simulink model "Subsystem1"  (R2023b)
settings: Solver=FixedStepAuto  StartTime=0.0  StopTime=10.0  FixedStep=5e-7  RelTol=1e-3
libraries: spsMosfetLib x6, spsDCVoltageSourceLib x1, spsPermanentMagnetSynchronousMachineLib x1, sps_lib x1
settings Model: Creator=LZQ  LastModifiedBy=LZQ
settings SolverCC: AllowMultiTaskInputOutput=on  ConcurrentTasks=on
settings DataIOCC: SaveOutput=off  SaveTime=off

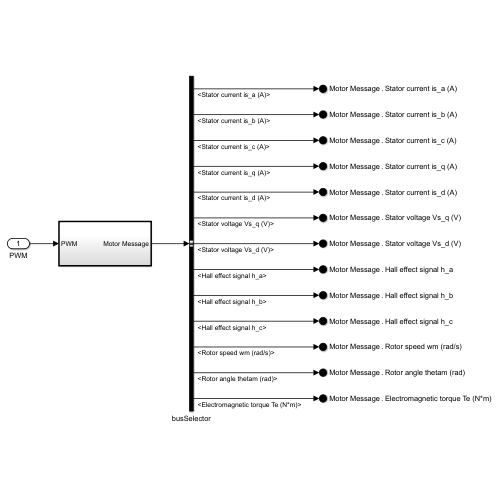
[thumbnail: Simulink's stored preview of the top-level diagram]
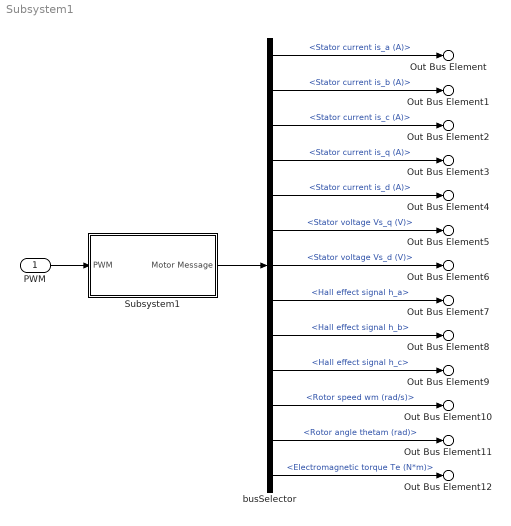
== system Subsystem1 ==
  PWM : Inport  OutDataTypeStr=double  PortDimensions=6  SampleTime=0
  Subsystem1 : Subsystem  TreatAsAtomicUnit=on
  busSelector : BusSelector  OutputSignals=Stator current is_a (A),Stator current is_b (A),Stator current is_c (A),Stator current is_q (A),Stator current is_d (A),Stator voltage Vs_q (V),Stator voltage Vs_d (V),Hall effect signal h_a,Hall effect signal h_b,Hall effect signal h_c,Rotor speed wm (rad/s),Rotor angle thetam (rad),Electromagnetic torque Te (N*m)
  Out Bus Element : Outport  PortName=Motor Message  Element=Stator current is_a (A)
  Out Bus Element1 : Outport  PortName=Motor Message  Element=Stator current is_b (A)
  Out Bus Element2 : Outport  PortName=Motor Message  Element=Stator current is_c (A)
  Out Bus Element3 : Outport  PortName=Motor Message  Element=Stator current is_q (A)
  Out Bus Element4 : Outport  PortName=Motor Message  Element=Stator current is_d (A)
  Out Bus Element5 : Outport  PortName=Motor Message  Element=Stator voltage Vs_q (V)
  Out Bus Element6 : Outport  PortName=Motor Message  Element=Stator voltage Vs_d (V)
  Out Bus Element7 : Outport  PortName=Motor Message  Element=Hall effect signal h_a
  Out Bus Element8 : Outport  PortName=Motor Message  Element=Hall effect signal h_b
  Out Bus Element9 : Outport  PortName=Motor Message  Element=Hall effect signal h_c
  Out Bus Element10 : Outport  PortName=Motor Message  Element=Rotor speed wm (rad/s)
  Out Bus Element11 : Outport  PortName=Motor Message  Element=Rotor angle thetam (rad)
  Out Bus Element12 : Outport  PortName=Motor Message  Element=Electromagnetic torque Te (N*m)
  wires:
  busSelector/4 -> Out Bus Element3/1  "<Stator current is_q (A)>"
  PWM/1 -> Subsystem1/1(PWM)
  busSelector/2 -> Out Bus Element1/1  "<Stator current is_b (A)>"
  Subsystem1/1(Motor Message) -> busSelector/1
  busSelector/1 -> Out Bus Element/1  "<Stator current is_a (A)>"
  busSelector/3 -> Out Bus Element2/1  "<Stator current is_c (A)>"
  busSelector/5 -> Out Bus Element4/1  "<Stator current is_d (A)>"
  busSelector/6 -> Out Bus Element5/1  "<Stator voltage Vs_q (V)>"
  busSelector/7 -> Out Bus Element6/1  "<Stator voltage Vs_d (V)>"
  busSelector/8 -> Out Bus Element7/1  "<Hall effect signal h_a>"
  busSelector/9 -> Out Bus Element8/1  "<Hall effect signal h_b>"
  busSelector/10 -> Out Bus Element9/1  "<Hall effect signal h_c>"
  busSelector/11 -> Out Bus Element10/1  "<Rotor speed wm (rad/s)>"
  busSelector/12 -> Out Bus Element11/1  "<Rotor angle thetam (rad)>"
  busSelector/13 -> Out Bus Element12/1  "<Electromagnetic torque Te (N*m)>"

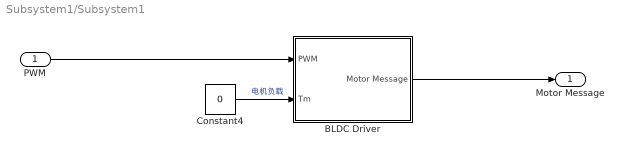
== system Subsystem1/Subsystem1 ==
  PWM : Inport
  BLDC Driver : Subsystem
  Constant4 : Constant  Value=0
  Motor Message : Outport
  wires:
  BLDC Driver/1(Motor Message) -> Motor Message/1
  PWM/1 -> BLDC Driver/1(PWM)
  Constant4/1 -> BLDC Driver/2(Tm)  "电机负载"

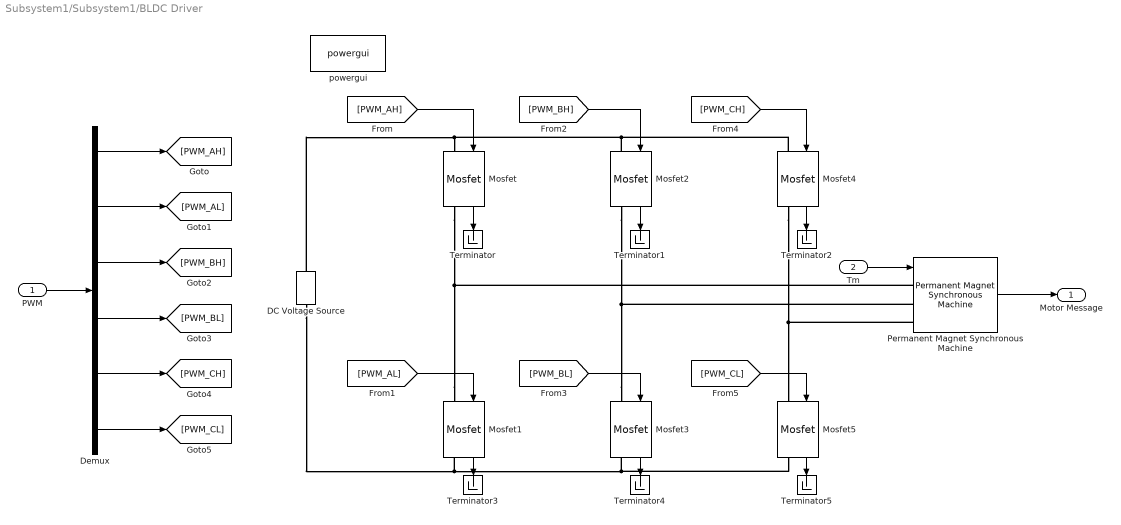
== system Subsystem1/Subsystem1/BLDC Driver ==
  PWM : Inport
  Tm : Inport  Port=2
  DC Voltage Source : spsDCVoltageSourceLib/DC Voltage Source  Amplitude=100  Measurements=Voltage
  Demux : Demux  Outputs=6
  Mosfet{,1..5} (6 alike) : spsMosfetLib/Mosfet  Ron=0.1  Lon=0  Rd=0.01  Vfd=0  IC=0  Rs=1e5  Cs=inf  Measurements=on
  Permanent Magnet Synchronous Machine : spsPermanentMagnetSynchronousMachineLib/Permanent Magnet Synchronous Machine  NbPhases=3  FluxDistribution=Sinusoidal  RotorType=Round  MechanicalLoad=Torque Tm  PresetModel=No  ShowDetailedParameters=on  MeasurementBus=off  Resistance=0.0485  Inductance=8.5e-3  dqInductances=[8.5e-3,8.5e-3]  La=0.000395  MachineConstant=Flux linkage established by magnets (V.s)  Flux=0.1194  VoltageCst=86.6271  TorqueCst=0.7164  Flat=120  Mechanical=[0.0027 0.0004924 4 0]  PolePairs=4  InitialConditions=[0,0, 0,0]  InitialConditions5ph=[0 0 0 0 0 0]  RefAngle=90 degrees behind phase A axis (modified Park)  IterativeDiscreteModel=Trapezoidal non iterative  TsBlock=-1  TsPowergui=0
  Terminator{,1..5} (6 alike) : Terminator
  powergui : sps_lib/powergui  Priority=1  SimulationMode=Discrete  SampleTime=5e-7  frequency=60  Iterations=50  frequencyindice=0  Pbase=100e6  ErrMax=1e-4  UnitsV=kV  UnitsW=MW  buscounter=0  FunctionMessages=off  echomessages=off  EnableUseOfTLC=off  CurrentSourceSwitches=off  DisableSnubberDevices=off  DisableRonSwitches=off  DisableVfSwitches=off  DisplayEquations=off  AutomaticDiscreteSolvers=off  SolverType=Tustin/Backward Euler (TBE)  Interpol=off  ExternalGateDelay=off  methode=off  Ts=100  x0status=blocks  SPID=on  SwTol=0  HookPort=off  NonlinearTolerance=1e-4  nMaxIteration=100  ContinueOnMaxIteration=off  RestoreLinks=warning  ResistiveCurrentMeasurement=off  Frange=[0:2:500]  Ylog=off  Xlog=on  ShowGrid=off  save=off  variable=ZData  structure=0  ZoomFFT=off  StartTime=0.0  cycles=1  DisplayStyle=1  fundamental=60  FreqAxis=off  MaxFrequency=1000  frequencyindicesteady=1  RmsSteady=1  display=off
  Motor Message : Outport
  wires:
  Tm/1 -> Permanent Magnet Synchronous Machine/1
  Permanent Magnet Synchronous Machine/1 -> Motor Message/1
  Demux/6 -> [PWM_CL]
  Demux/5 -> [PWM_CH]
  Demux/4 -> [PWM_BL]
  Demux/3 -> [PWM_BH]
  Demux/2 -> [PWM_AL]
  Demux/1 -> [PWM_AH]
  PWM/1 -> Demux/1
  [PWM_CL] -> Mosfet5/1
  [PWM_CH] -> Mosfet4/1
  [PWM_AL] -> Mosfet1/1
  [PWM_BL] -> Mosfet3/1
  [PWM_BH] -> Mosfet2/1
  Mosfet5/1 -> Terminator5/1
  Mosfet3/1 -> Terminator4/1
  Mosfet1/1 -> Terminator3/1
  Mosfet4/1 -> Terminator2/1
  Mosfet2/1 -> Terminator1/1
  Mosfet/1 -> Terminator/1
  [PWM_AH] -> Mosfet/1
  connections:
  Mosfet1/RConn1 -- Mosfet3/RConn1 -- Mosfet5/RConn1 -- DC Voltage Source/LConn1
  Mosfet/LConn1 -- Mosfet2/LConn1 -- Mosfet4/LConn1 -- DC Voltage Source/RConn1
  Permanent Magnet Synchronous Machine/LConn3 -- Mosfet5/LConn1 -- Mosfet4/RConn1
  Mosfet1/LConn1 -- Permanent Magnet Synchronous Machine/LConn1 -- Mosfet/RConn1
  Mosfet3/LConn1 -- Permanent Magnet Synchronous Machine/LConn2 -- Mosfet2/RConn1
